simulink library "DCCI_lib"  (Simulink 7.5)
settings: Solver=ode45  StartTime=0.0  StopTime=10.0  RelTol=1e-3
undefined symbols (not defined in the file or in its folder): DCDCStsTyp, p_bool_True_M, p_single_Zero_M
libraries: BaseOperationLib_Browser x6, PES_CZ_FAW x2, simulink x1
settings Model: Creator=wuaibin  LastModifiedBy=wuaibin

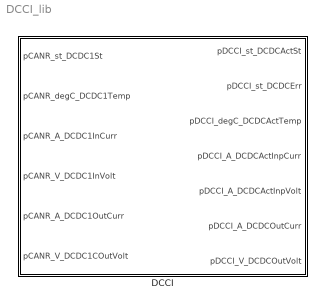
== system DCCI_lib ==
  DCCI : Subsystem  TreatAsAtomicUnit=on

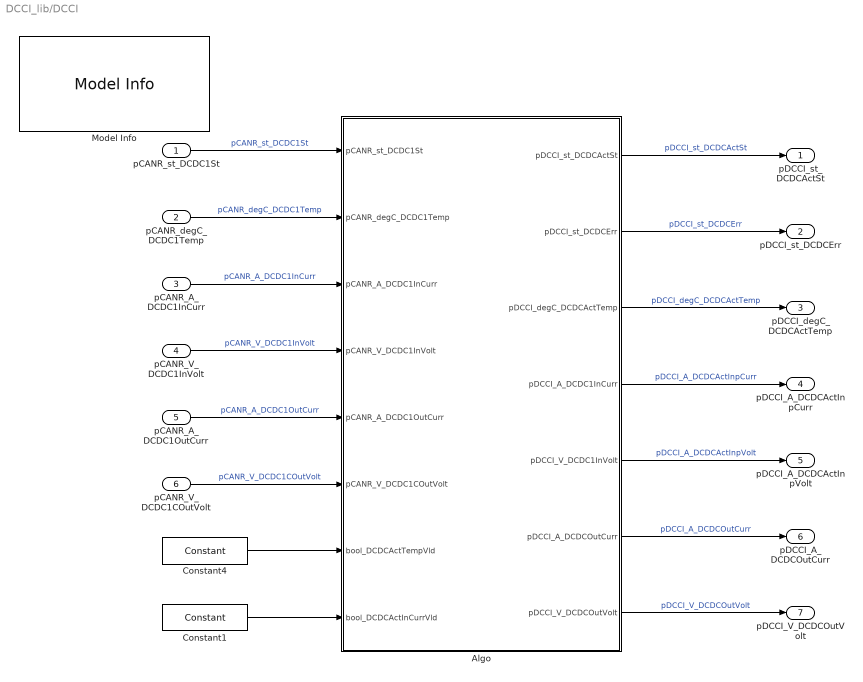
== system DCCI_lib/DCCI ==
  pCANR_st_DCDC1St : Inport  OutDataType=fixdt(1, 16)  OutScaling=2^0
  pCANR_degC_DCDC1Temp : Inport  Port=2  OutDataType=fixdt(1, 16)  OutScaling=2^0
  pCANR_A_DCDC1InCurr : Inport  Port=3  OutDataType=fixdt(1, 16)  OutScaling=2^0
  pCANR_V_DCDC1InVolt : Inport  Port=4  OutDataType=fixdt(1, 16)  OutScaling=2^0
  pCANR_A_DCDC1OutCurr : Inport  Port=5
  pCANR_V_DCDC1COutVolt : Inport  Port=6
  Algo : Subsystem
  Constant1 : BaseOperationLib_Browser/Sources&Sinks/Constant  Value=p_bool_True_M  OutMin=[]  OutMax=[]  OutDataTypeMode=boolean  OutDataType=fixdt(1, 16)  ConRadixGroup=Use specified scaling  OutScaling=2^0  OutDataTypeStr=boolean
  Constant4 : BaseOperationLib_Browser/Sources&Sinks/Constant  Value=p_bool_True_M  OutMin=[]  OutMax=[]  OutDataTypeMode=boolean  OutDataType=fixdt(1, 16)  ConRadixGroup=Use specified scaling  OutScaling=2^0  OutDataTypeStr=boolean
  Model Info : simulink/Model-Wide Utilities/Model Info  SystemSampleTime=-1  InitialBlockCM=None  BlockCM=None  Frame=on  DisplayStringWithTags=Model Info\nCreated: %<Created>\nCreator: zhangqiang  HorizontalTextAlignment=Center  LeftAlignmentValue=0.5  SourceBlockDiagram=HQEV_HCU  TagMaxNumber=20
  pDCCI_st_DCDCActSt : Outport  OutDataType=fixdt(1, 16)  OutScaling=2^0
  pDCCI_st_DCDCErr : Outport  Port=2  OutDataType=fixdt(1, 16)  OutScaling=2^0
  pDCCI_degC_DCDCActTemp : Outport  Port=3  OutDataType=fixdt(1, 16)  OutScaling=2^0
  pDCCI_A_DCDCActInpCurr : Outport  Port=4  OutDataType=fixdt(1, 16)  OutScaling=2^0
  pDCCI_A_DCDCActInpVolt : Outport  Port=5
  pDCCI_A_DCDCOutCurr : Outport  Port=6
  pDCCI_V_DCDCOutVolt : Outport  Port=7
  wires:
  Constant1/1 -> Algo/8(bool_DCDCActInCurrVld)
  Constant4/1 -> Algo/7(bool_DCDCActTempVld)
  pCANR_V_DCDC1InVolt/1 -> Algo/4(pCANR_V_DCDC1InVolt)  "pCANR_V_DCDC1InVolt"
  Algo/2(pDCCI_st_DCDCErr) -> pDCCI_st_DCDCErr/1  "pDCCI_st_DCDCErr"
  pCANR_st_DCDC1St/1 -> Algo/1(pCANR_st_DCDC1St)  "pCANR_st_DCDC1St"
  Algo/1(pDCCI_st_DCDCActSt) -> pDCCI_st_DCDCActSt/1  "pDCCI_st_DCDCActSt"
  pCANR_degC_DCDC1Temp/1 -> Algo/2(pCANR_degC_DCDC1Temp)  "pCANR_degC_DCDC1Temp"
  Algo/3(pDCCI_degC_DCDCActTemp) -> pDCCI_degC_DCDCActTemp/1  "pDCCI_degC_DCDCActTemp"
  pCANR_A_DCDC1InCurr/1 -> Algo/3(pCANR_A_DCDC1InCurr)  "pCANR_A_DCDC1InCurr"
  Algo/4(pDCCI_A_DCDC1InCurr) -> pDCCI_A_DCDCActInpCurr/1  "pDCCI_A_DCDCActInpCurr"
  pCANR_V_DCDC1COutVolt/1 -> Algo/6(pCANR_V_DCDC1COutVolt)  "pCANR_V_DCDC1COutVolt"
  pCANR_A_DCDC1OutCurr/1 -> Algo/5(pCANR_A_DCDC1OutCurr)  "pCANR_A_DCDC1OutCurr"
  Algo/5(pDCCI_V_DCDC1InVolt) -> pDCCI_A_DCDCActInpVolt/1  "pDCCI_A_DCDCActInpVolt"
  Algo/7(pDCCI_V_DCDCOutVolt) -> pDCCI_V_DCDCOutVolt/1  "pDCCI_V_DCDCOutVolt"
  Algo/6(pDCCI_A_DCDCOutCurr) -> pDCCI_A_DCDCOutCurr/1  "pDCCI_A_DCDCOutCurr"

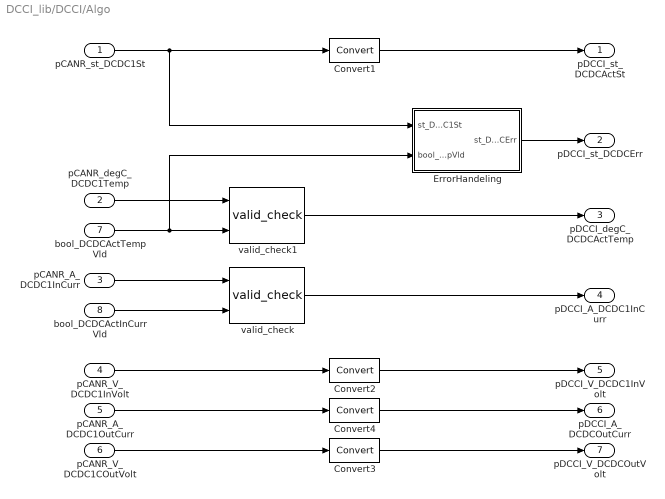
== system DCCI_lib/DCCI/Algo ==
  pCANR_st_DCDC1St : Inport  OutDataType=fixdt(1, 16)  OutScaling=2^0
  pCANR_degC_DCDC1Temp : Inport  Port=2  OutDataType=fixdt(1, 16)  OutScaling=2^0
  pCANR_A_DCDC1InCurr : Inport  Port=3  OutDataType=fixdt(1, 16)  OutScaling=2^0
  pCANR_V_DCDC1InVolt : Inport  Port=4
  pCANR_A_DCDC1OutCurr : Inport  Port=5
  pCANR_V_DCDC1COutVolt : Inport  Port=6
  bool_DCDCActTempVld : Inport  Port=7  OutDataType=fixdt(1, 16)  OutScaling=2^0
  bool_DCDCActInCurrVld : Inport  Port=8  OutDataType=fixdt(1, 16)  OutScaling=2^0
  Convert{1..4} (4 alike) : DataTypeConversion  OutDataType=fixdt(1, 16)  OutScaling=2^0
  ErrorHandeling : Subsystem
  valid_check : PES_CZ_FAW/Discontinuities/valid_check  SystemSampleTime=-1  init=0
  valid_check1 : PES_CZ_FAW/Discontinuities/valid_check  SystemSampleTime=-1  init=pDCCI_degC_DcDcActInitTemp_C
  pDCCI_st_DCDCActSt : Outport  OutDataType=fixdt(1, 16)  OutScaling=2^0
  pDCCI_st_DCDCErr : Outport  Port=2  OutDataType=fixdt(1, 16)  OutScaling=2^0
  pDCCI_degC_DCDCActTemp : Outport  Port=3  OutDataType=fixdt(1, 16)  OutScaling=2^0
  pDCCI_A_DCDC1InCurr : Outport  Port=4  OutDataType=fixdt(1, 16)  OutScaling=2^0
  pDCCI_V_DCDC1InVolt : Outport  Port=5
  pDCCI_A_DCDCOutCurr : Outport  Port=6
  pDCCI_V_DCDCOutVolt : Outport  Port=7
  wires:
  Convert4/1 -> pDCCI_A_DCDCOutCurr/1
  Convert3/1 -> pDCCI_V_DCDCOutVolt/1
  Convert2/1 -> pDCCI_V_DCDC1InVolt/1
  Convert1/1 -> pDCCI_st_DCDCActSt/1
  pCANR_V_DCDC1InVolt/1 -> Convert2/1
  pCANR_st_DCDC1St/1 -> Convert1/1, ErrorHandeling/1(st_DCDC1St)
  pCANR_A_DCDC1InCurr/1 -> valid_check/1
  bool_DCDCActInCurrVld/1 -> valid_check/2
  valid_check/1 -> pDCCI_A_DCDC1InCurr/1
  pCANR_degC_DCDC1Temp/1 -> valid_check1/1
  bool_DCDCActTempVld/1 -> valid_check1/2, ErrorHandeling/2(bool_DCDCActTempVld)
  valid_check1/1 -> pDCCI_degC_DCDCActTemp/1
  ErrorHandeling/1(st_DCDCErr) -> pDCCI_st_DCDCErr/1
  pCANR_V_DCDC1COutVolt/1 -> Convert3/1
  pCANR_A_DCDC1OutCurr/1 -> Convert4/1

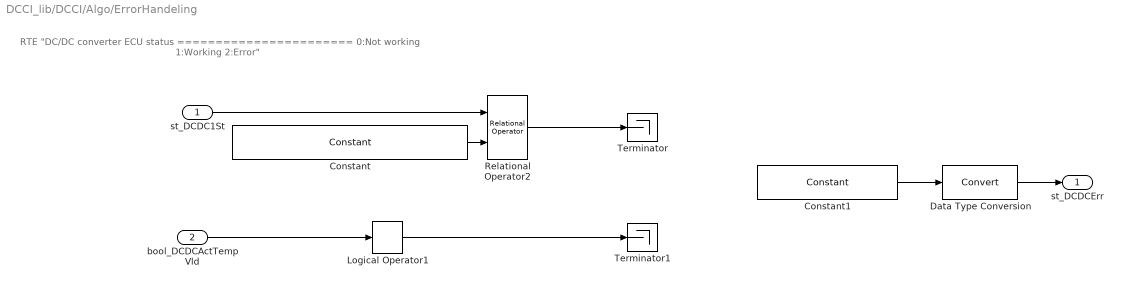
== system DCCI_lib/DCCI/Algo/ErrorHandeling ==
  note: RTE "DC/DC converter ECU status
      | =======================
      | 0:Not working
      | 1:Working
      | 2:Error"
  st_DCDC1St : Inport  OutDataType=fixdt(1, 16)  OutScaling=2^0
  bool_DCDCActTempVld : Inport  Port=2  OutDataType=fixdt(1, 16)  OutScaling=2^0
  Constant : BaseOperationLib_Browser/Sources&Sinks/Constant  Value=uint8(DCDCStsTyp.DCDC_CANTIMEOUT_ERR)  OutMin=[]  OutMax=[]  OutDataType=fixdt(1, 16)  ConRadixGroup=Use specified scaling  OutScaling=2^0  OutDataTypeStr=Inherit: Inherit via back propagation
  Constant1 : BaseOperationLib_Browser/Sources&Sinks/Constant  Value=p_single_Zero_M  OutMin=[]  OutMax=[]  OutDataType=fixdt(1, 16)  ConRadixGroup=Use specified scaling  OutScaling=2^0  OutDataTypeStr=Inherit: Inherit from 'Constant value'
  Data Type Conversion : DataTypeConversion  OutDataType=fixdt(1, 16)  OutScaling=2^0
  Logical Operator1 : BaseOperationLib_Browser/Logic Operations Changed/Logical Operator  Operator=NOT  Inputs=2  AllPortsSameDT=on  OutDataTypeMode=Specify via dialog  LogicDataType=PDT_Bool  OutDataTypeStr=PDT_Bool
  Relational Operator2 : BaseOperationLib_Browser/Logic Operations Changed/Relational Operator  Operator===  InputSameDT=on  LogicOutDataTypeMode=Specify via dialog  LogicDataType=PDT_Bool  OutDataTypeStr=PDT_Bool
  Terminator : Terminator
  Terminator1 : Terminator
  st_DCDCErr : Outport  OutDataType=fixdt(1, 16)  OutScaling=2^0
  wires:
  Data Type Conversion/1 -> st_DCDCErr/1
  Logical Operator1/1 -> Terminator1/1
  Relational Operator2/1 -> Terminator/1
  Constant1/1 -> Data Type Conversion/1
  st_DCDC1St/1 -> Relational Operator2/1
  Constant/1 -> Relational Operator2/2
  bool_DCDCActTempVld/1 -> Logical Operator1/1
